simulink library "LIB_ROT"  (Simulink 8.8)
settings: Solver=ode45  StartTime=0.0  StopTime=10.0  RelTol=1e-3  EnableMultiTasking=on
undefined symbols (not defined in the file): EARTHstates
settings Model: Creator=alger  LastModifiedBy=alger

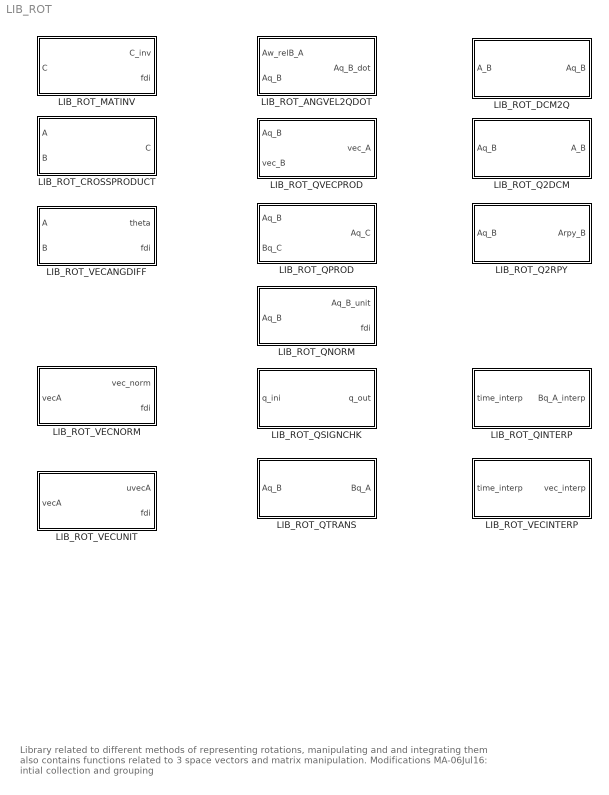
== system LIB_ROT ==
  note: Library related to different methods of representing rotations, manipulating and and integrating them
      | also contains functions related to 3 space vectors and matrix manipulation.
      |
      | Modifications
      | MA-06Jul16: intial collection and grouping
  LIB_ROT_ANGVEL2QDOT : Subsystem  TreatAsAtomicUnit=on  mask(Compute Quaternion derivative from angular velocity){}
      mask help:
      | Compute quaternion derivative using method outlined in GEI720 course notes.
      |
      | Inputs:
      |   Aw_relB_A:  Angular velocity of frame A, relative to B, expressed in A (rad/s).
      |   Aq_B:  Current attitude of A relative to B in quaternion.
      |
      | Outputs:
      |   Aq_B_dot:  Quaternion derivative of frame A in frame B.
      |
      | uses angvel2qdot function()
  LIB_ROT_CROSSPRODUCT : Subsystem  TreatAsAtomicUnit=on  mask(Cross product){}
      mask help:
      | Computes cross product of two 3 element vectors
      |
      | Inputs:
      | A first 3 element vector
      | B second 3 element vector
      |
      | Outputs:
      | C resulting 3 element cross product.
      |
      | uses cross() matlab function
  LIB_ROT_DCM2Q : Subsystem  TreatAsAtomicUnit=on  mask(transforms Direction Cosine Matrix to a quaternion){}
      mask help:
      | This function converts a DCM to a quaternion
      |
      | Inputs:
      |   A_B: DCM that relates a vector in frame B to the same vector in frame A
      |
      | Outputs:
      |   Aq_B: an equivlant quaternion that relates a vector in frame B to a the same vector in frame A
      |
      | uses dcm2q() function
  "LIB_ROT_MATINV " : Subsystem  TreatAsAtomicUnit=on  mask(Matrix Inverse){tol=0}
      mask prompts: tol "Near zero tolerence"
      mask help:
      | Computes the inverse of a matrix using by checking the determinant first. If the determinant is greater than a specified tolerence the matrix is inverted
      |
      | Inputs:
      | C: a square matrix to invert
      |
      | Outputs:
      | C_inv: the inverse of C if it is possible to compute if not a similarly sized zero matrix is returned
      | fdi: flag that indicates inverting the matrix was not possible 0: no issue 1: not invertable with given tolerance
      |
      | uses the matinv() function,
  LIB_ROT_Q2DCM : Subsystem  TreatAsAtomicUnit=on  mask(Transforms a quaternion to a direction cosine matrix){}
      mask help:
      | this function converts a quaternion to a direction cosine matrix
      |
      | Inputs:
      |   Aq_B: quaternion that relates a vector in frame B to the same vector in frame A
      |
      | Outputs:
      |  A_B: an equivilant DCM that relates a vector in frame B to the same vector in frame A
      |
      | uses q2dcm() function
  LIB_ROT_Q2RPY : Subsystem  TreatAsAtomicUnit=on  mask(Converts Quaternion to 3-2-1 euler rotation){}
      mask help:
      | This function checks if the quaternion has a positive scalar component and returns the positive equivalent quaternion if it is not.
      |
      | Inputs:
      |   Aq_B: input quaternion
      |
      | Outputs:
      |   Arpy_B: roll pitch and yaw in a vector [roll; pitch; yaw];
      |
      | uses q2rpy() function
  LIB_ROT_QINTERP : Subsystem  TreatAsAtomicUnit=on  mask(interpolates quaternion values found in a supplied table){time_start=|, time_step=0, Bq_A_ref=|}
      mask time_start=|
      | [     0;
      |    180;
      |    360;
      |    540;
      |    720]
      mask Bq_A_ref=|
      | [        0.659846541112867,      0.000660604589589575,      0.000553547923653578,          0.75139989311129;
      |          0.654901001122464,       0.00066423707317091,      0.000549196429684912,         0.755714189294595;
      |          0.649927253531624,      0.000667840948371602,      0.000544821276719665,         0.759995935696425;
      |          0.644925512567267,      0.000671416059940447,       0.00054042265319099,         0.764244947895423;
      |          0.639895993662054,      0.000674962253865271,      0.000536000748543387,         0.768461042880123]
      mask prompts: Bq_A_ref "vector of quaternions [n x 4]"
      mask help:
      | this function computes the interpolated value of a quaternion for a given time
      |
      | Inputs
      | time_interp: time to compute the interpolation for
      |
      | Outputs
      | Bq_A_interp: vector interpolated at time_interp
      |
      | uses vecinterp() function
  LIB_ROT_QNORM : Subsystem  TreatAsAtomicUnit=on  mask(Normalize Quaternion){zero_tol=0}
      mask prompts: zero_tol "near zero tolerance"
      mask help:
      | This function computes the norm of a quaternion using method
      | outlined in section 5.6. of Kuipers 1999
      |
      | Inputs:
      |   Aq_B: Quaternion representing rotation of frame B to frame A
      |   tol:  tolerance to use on quaternion unit length if not specified 10e-9 is used
      |
      | Outputs:
      |   Aq_B_unit: unit quaternion of Aq_B
      |   fdi: 1 indicates that unit length computed is less than tolerance
      |
      | uses qnorm()function
  LIB_ROT_QPROD : Subsystem  TreatAsAtomicUnit=on  mask(Combines quaternion frame rotations into a single quaternion){}
      mask help:
      | Relates one frame to another through an intermediary frame
      | i.e. Aq_C = Aq_B x Bq_C.
      |
      | Inputs
      |   Aq_B: quaternion representing the rotation of a vector in frame B to frame A
      |   Bq_C: quaternion representing the rotation of a vector in frame C to frame B
      |
      | Outputs
      |   Aq_C quaternion representing the rotation of a vector in frame C to frame A
      |
      | uses qprod() function
  LIB_ROT_QSIGNCHK : Subsystem  TreatAsAtomicUnit=on  mask(Ensures quaterion has a positive scalar component){tol=0}
      mask prompts: tol "near zero tolerance"
      mask help:
      | This function checks if the quaternion has a positive scalar component and returns the positive equivalent quaternion if it is not.
      |
      | Inputs:
      |   q_in: input quaternion
      |
      | Outputs:
      |   q_out: output quaternion;
      |
      | uses qsignchck() function
  LIB_ROT_QTRANS : Subsystem  TreatAsAtomicUnit=on  mask(computes transposed quaternion){}
      mask help:
      | This function computes the transposed quaterion (quaternion inverse of a unit quaternion), it also ensures the returned value has a positive scalar component.
      |
      | Inputs:
      |   q_in: input quaternion
      |
      | Outputs:
      |   q_out: output quaternion;
      |
      | uses qsignchck() function
  LIB_ROT_QVECPROD : Subsystem  TreatAsAtomicUnit=on  mask(Rotate a vector by quaternion){}
      mask help:
      | Discription:
      |  This function rotates a vector by the supplied rotation described by
      |  Aq_B i.e. vec_A = Aq_B x vec_B.
      |  this function follows the reuslt shown in section 5.8 of Kuiperss 1999.
      |
      | Inputs
      |   Aq_B: quaternion representing the rotation of a vector in frame B to frame A
      |   vec_B: vector expressed in frame B
      |
      | Outputs
      |   vec_A vector expressed in frame A
      |
      | uses qvecprod() function
  LIB_ROT_VECANGDIFF : Subsystem  TreatAsAtomicUnit=on  mask(Computes the angle between two vectors){zero_tol=0}
      mask prompts: zero_tol "near zero tolerance"
      mask help:
      | Computes the angle between two vectors
      |
      | Inputs:
      | A first 3 element vector
      | B second3 element vector
      |
      | Outputs:
      | theta: minimum angle between the two vectors
      | fdi: an indication that one of the two vectors is smaller than the given tolerance
      |
      |
      |
      | uses vecangdiff() matlab function
  LIB_ROT_VECINTERP : Subsystem  TreatAsAtomicUnit=on  mask(interpolates vector values found in a supplied table){time_start=EARTHstates.time_relJDepoch_TAI_days_start, time_step=EARTHstates.time_relJDepoch_TAI_days_step, vec_ref=EARTHstates.BCBFw_relCEL_BCBF}
      mask prompts: time_start "time_start[n]"; vec_ref "vec_ref [n x 3]"
      mask help:
      | this function computes the interpolated value of a vector for a given time
      |
      | Inputs
      | time_interp: time to compute the interpolation for
      |
      | Outputs
      | vec_interp: vector interpolated at time_interp
      |
      | uses qinterp() function
  LIB_ROT_VECNORM : Subsystem  TreatAsAtomicUnit=on  mask(Computes the 2 space norm of a vector){zero_tol=0}
      mask prompts: zero_tol "near zero tolerance"
      mask help:
      | Computes the 2 space norm of a vector
      |
      | Inputs:
      | vecA first 3 element vector
      |
      |
      | Outputs:
      | norm: : the norm of the vector
      | fdi: an indication that one of the two vectors is smaller than the given tolerance
      |
      |
      |
      | uses vecangdiff() matlab function
  LIB_ROT_VECUNIT : Subsystem  TreatAsAtomicUnit=on  mask(Computes the unit vector for a given vector){zero_tol=0}
      mask prompts: zero_tol "near zero tolerance"
      mask help:
      | Computes the unit vector for a given vector
      |
      | Inputs:
      | vecA first 3 element vector
      |
      |
      | Outputs:
      | uvecA  resulting unit vector
      | fdi: an indication that one of the two vectors is smaller than the given tolerance
      |
      |
      |
      | uses vecangdiff() matlab function

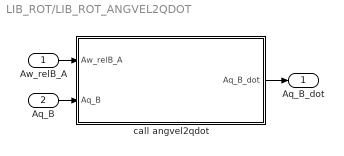
== system LIB_ROT/LIB_ROT_ANGVEL2QDOT ==
  Aw_relB_A : Inport  PortDimensions=3
  Aq_B : Inport  Port=2  PortDimensions=4
  call angvel2qdot : MATLAB Function  TreatAsAtomicUnit=on
  Aq_B_dot : Outport  PortDimensions=4
  wires:
  Aw_relB_A/1 -> call angvel2qdot/1(Aw_relB_A)
  Aq_B/1 -> call angvel2qdot/2(Aq_B)
  call angvel2qdot/1(Aq_B_dot) -> Aq_B_dot/1

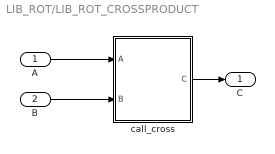
== system LIB_ROT/LIB_ROT_CROSSPRODUCT ==
  A : Inport  PortDimensions=3
  B : Inport  Port=2  PortDimensions=3
  call_cross : MATLAB Function  TreatAsAtomicUnit=on
  C : Outport  PortDimensions=3
  wires:
  call_cross/1(C) -> C/1
  B/1 -> call_cross/2(B)
  A/1 -> call_cross/1(A)

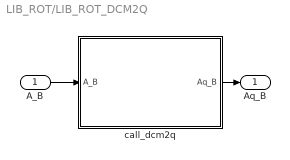
== system LIB_ROT/LIB_ROT_DCM2Q ==
  A_B : Inport  PortDimensions=[3,3]
  "call_dcm2q " : MATLAB Function  TreatAsAtomicUnit=on
  Aq_B : Outport  PortDimensions=4
  wires:
  A_B/1 -> "call_dcm2q "/1(A_B)
  "call_dcm2q "/1(Aq_B) -> Aq_B/1

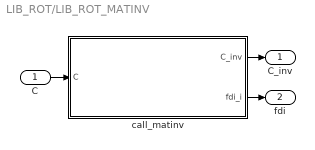
== system LIB_ROT/LIB_ROT_MATINV  ==
  C : Inport
  call_matinv : MATLAB Function  TreatAsAtomicUnit=on
  C_inv : Outport
  fdi : Outport  Port=2
  wires:
  call_matinv/1(C_inv) -> C_inv/1
  C/1 -> call_matinv/1(C)
  call_matinv/2(fdi_i) -> fdi/1

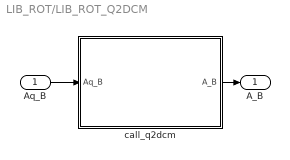
== system LIB_ROT/LIB_ROT_Q2DCM ==
  Aq_B : Inport  PortDimensions=4
  "call_q2dcm " : MATLAB Function  TreatAsAtomicUnit=on
  A_B : Outport  PortDimensions=[3,3]
  wires:
  "call_q2dcm "/1(A_B) -> A_B/1
  Aq_B/1 -> "call_q2dcm "/1(Aq_B)

== system LIB_ROT/LIB_ROT_Q2RPY ==
  Aq_B : Inport  PortDimensions=4
  "call_q2rpy " : MATLAB Function  TreatAsAtomicUnit=on
  Arpy_B : Outport  PortDimensions=3
  wires:
  Aq_B/1 -> "call_q2rpy "/1(Aq_B)
  "call_q2rpy "/1(Arpy_B) -> Arpy_B/1

== system LIB_ROT/LIB_ROT_QINTERP ==
  time_interp : Inport  PortDimensions=1
  "call_qinterp " : MATLAB Function  TreatAsAtomicUnit=on
  Bq_A_interp : Outport  PortDimensions=4
  wires:
  time_interp/1 -> "call_qinterp "/1(time_interp)
  "call_qinterp "/1(Bq_A_interp) -> Bq_A_interp/1

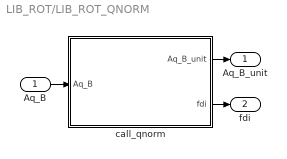
== system LIB_ROT/LIB_ROT_QNORM ==
  Aq_B : Inport  PortDimensions=4
  "call_qnorm " : MATLAB Function  TreatAsAtomicUnit=on
  Aq_B_unit : Outport  PortDimensions=4
  fdi : Outport  Port=2  PortDimensions=1
  wires:
  "call_qnorm "/2(fdi) -> fdi/1
  "call_qnorm "/1(Aq_B_unit) -> Aq_B_unit/1
  Aq_B/1 -> "call_qnorm "/1(Aq_B)

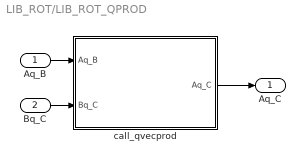
== system LIB_ROT/LIB_ROT_QPROD ==
  Aq_B : Inport  PortDimensions=4
  Bq_C : Inport  Port=2  PortDimensions=4
  "call_qvecprod  " : MATLAB Function  TreatAsAtomicUnit=on
  Aq_C : Outport  PortDimensions=4
  wires:
  Bq_C/1 -> "call_qvecprod  "/2(Bq_C)
  "call_qvecprod  "/1(Aq_C) -> Aq_C/1
  Aq_B/1 -> "call_qvecprod  "/1(Aq_B)

== system LIB_ROT/LIB_ROT_QSIGNCHK ==
  q_ini : Inport  PortDimensions=4
  "call_qsignchk " : MATLAB Function  TreatAsAtomicUnit=on
  q_out : Outport  PortDimensions=4
  wires:
  q_ini/1 -> "call_qsignchk "/1(q_in)
  "call_qsignchk "/1(q_out) -> q_out/1

== system LIB_ROT/LIB_ROT_QTRANS ==
  Aq_B : Inport  PortDimensions=4
  "call_qtrans " : MATLAB Function  TreatAsAtomicUnit=on
  Bq_A : Outport  PortDimensions=4
  wires:
  "call_qtrans "/1(Bq_A) -> Bq_A/1
  Aq_B/1 -> "call_qtrans "/1(Aq_B)

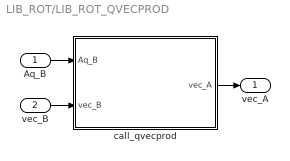
== system LIB_ROT/LIB_ROT_QVECPROD ==
  Aq_B : Inport  PortDimensions=4
  vec_B : Inport  Port=2  PortDimensions=3
  "call_qvecprod  " : MATLAB Function  TreatAsAtomicUnit=on
  vec_A : Outport  PortDimensions=3
  wires:
  Aq_B/1 -> "call_qvecprod  "/1(Aq_B)
  "call_qvecprod  "/1(vec_A) -> vec_A/1
  vec_B/1 -> "call_qvecprod  "/2(vec_B)

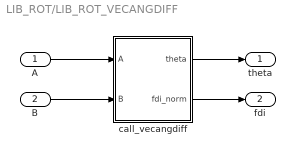
== system LIB_ROT/LIB_ROT_VECANGDIFF ==
  A : Inport  PortDimensions=3
  B : Inport  Port=2  PortDimensions=3
  call_vecangdiff : MATLAB Function  TreatAsAtomicUnit=on
  theta : Outport  PortDimensions=1
  fdi : Outport  Port=2  PortDimensions=1
  wires:
  A/1 -> call_vecangdiff/1(A)
  B/1 -> call_vecangdiff/2(B)
  call_vecangdiff/1(theta) -> theta/1
  call_vecangdiff/2(fdi_norm) -> fdi/1

== system LIB_ROT/LIB_ROT_VECINTERP ==
  time_interp : Inport  PortDimensions=1
  MATLAB Function : MATLAB Function  TreatAsAtomicUnit=on
  vec_interp : Outport  PortDimensions=3
  wires:
  MATLAB Function/1(vec_interp) -> vec_interp/1
  time_interp/1 -> MATLAB Function/1(time_interp)

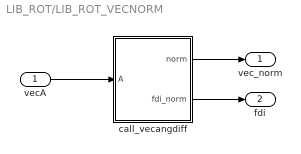
== system LIB_ROT/LIB_ROT_VECNORM ==
  vecA : Inport  PortDimensions=3
  call_vecangdiff : MATLAB Function  TreatAsAtomicUnit=on
  vec_norm : Outport  PortDimensions=1
  fdi : Outport  Port=2  PortDimensions=1
  wires:
  call_vecangdiff/2(fdi_norm) -> fdi/1
  call_vecangdiff/1(norm) -> vec_norm/1
  vecA/1 -> call_vecangdiff/1(A)

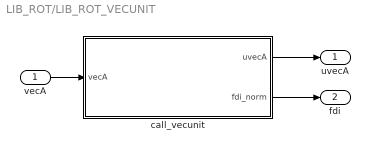
== system LIB_ROT/LIB_ROT_VECUNIT ==
  vecA : Inport  PortDimensions=3
  call_vecunit : MATLAB Function  TreatAsAtomicUnit=on
  uvecA : Outport  PortDimensions=3
  fdi : Outport  Port=2  PortDimensions=1
  wires:
  vecA/1 -> call_vecunit/1(vecA)
  call_vecunit/1(uvecA) -> uvecA/1
  call_vecunit/2(fdi_norm) -> fdi/1

== matlab function LIB_ROT_CROSSPRODUCT/call_cross ==
  data: A input double; C output double; B input double
function C = call_cross(A, B)
%#codegen
  C = crossmat(A) * B;
end

== matlab function LIB_ROT_MATINV /call_matinv ==
  data: C input double; C_inv output double; tol parameter double; fdi_i output double
function [C_inv, fdi_i] = call_matinv(C, tol)
  %#codegen
  [C_inv, fdi_i] = matinv(C, tol);
end

== matlab function LIB_ROT_ANGVEL2QDOT/call angvel2qdot ==
  data: Aw_relB_A input double; Aq_B_dot output double; Aq_B input double
function Aq_B_dot = call_angvel2qdot(Aw_relB_A, Aq_B)
  %#codegen
  Aq_B_dot = angvel2qdot(Aw_relB_A, Aq_B);
end

== matlab function LIB_ROT_QNORM/call_qnorm  ==
  data: Aq_B input double; Aq_B_unit output double; zero_tol parameter double; fdi output double
function [Aq_B_unit, fdi] = call_qnorm(Aq_B, zero_tol)
%#codegen
[Aq_B_unit, fdi] = qnorm(Aq_B, zero_tol);
end

== matlab function LIB_ROT_QSIGNCHK/call_qsignchk  ==
  data: q_in input double; q_out output double
function q_out  = call_qsignchk(q_in)
%#codegen
 [q_out] = qsignchk(q_in);
end

== matlab function LIB_ROT_QVECPROD/call_qvecprod  ==
  data: Aq_B input double; vec_A output double; vec_B input double
function vec_A  = call_qvecprod(Aq_B, vec_B)
  %#codegen
  
%   [vec_A] = qvecprod(qtrans(Aq_B), vec_B );
  [vec_A] = qvecprod(Aq_B, vec_B);
end

== matlab function LIB_ROT_QPROD/call_qvecprod  ==
  data: Aq_B input double; Aq_C output double; Bq_C input double
function Aq_C  = call_qprod(Aq_B, Bq_C)
  %#codegen
  
  [Aq_C] = qprod(Aq_B, Bq_C);
end

== matlab function LIB_ROT_QTRANS/call_qtrans  ==
  data: Aq_B input double; Bq_A output double
function Bq_A  = call_qtrans(Aq_B)
%#codegen
 Bq_A  = qtrans(Aq_B);
end

== matlab function LIB_ROT_Q2DCM/call_q2dcm  ==
  data: Aq_B input double; A_B output double
function A_B  = call_q2dcm(Aq_B)
%#codegen
 [ A_B ] = q2dcm(Aq_B);
end

== matlab function LIB_ROT_DCM2Q/call_dcm2q  ==
  data: Aq_B output double; A_B input double
function Aq_B  = call_dcm2q(A_B)
%#codegen
 [ Aq_B ] = dcm2q(A_B);
end

== matlab function LIB_ROT_Q2RPY/call_q2rpy  ==
  data: Aq_B input double; Arpy_B output double
function Arpy_B = call_q2rpy(Aq_B)
%#codegen
 [ Arpy_B ] = q2rpy(Aq_B);
end

== matlab function LIB_ROT_VECANGDIFF/call_vecangdiff ==
  data: A input double; theta output double; B input double; zero_tol parameter double; fdi_norm output double
function [theta, fdi_norm] = call_vecangdiff(A, B,zero_tol)
%#codegen
  [theta, fdi_norm] = vecangdiff(A, B, zero_tol);
end

== matlab function LIB_ROT_QINTERP/call_qinterp  ==
  data: time_start parameter double; Bq_A_interp output double size=4; time_step parameter double; Bq_A_ref parameter double; time_interp input double size=1
function Bq_A_interp  = call_qinterp(time_start, time_step, Bq_A_ref, time_interp)
%#codegen
[Bq_A_interp] = qinterp(time_start, time_step, Bq_A_ref, time_interp);
end

== matlab function LIB_ROT_VECINTERP/MATLAB Function ==
  data: time_start parameter double; vec_interp output double; time_step parameter double; vec_ref parameter double; time_interp input double size=1
function vec_interp = call_vecinterp( time_start, time_step, vec_ref, time_interp)
  %#codegen

    vec_interp = vecinterp(time_start, time_step, vec_ref, time_interp);

end

== matlab function LIB_ROT_VECNORM/call_vecangdiff ==
  data: A input double; norm output double; zero_tol parameter double; fdi_norm output double
function [norm, fdi_norm] = call_vecnorm(A,zero_tol)
%#codegen
  [norm, fdi_norm] = vecnorm(A, zero_tol);
end

== matlab function LIB_ROT_VECUNIT/call_vecunit ==
  data: vecA input double; uvecA output double; zero_tol parameter double; fdi_norm output double
function [uvecA, fdi_norm] = call_vecunit(vecA,zero_tol)
%#codegen
  [uvecA, fdi_norm] = vecunit(vecA, zero_tol);
end
